simulink model "simLab11"  (R2023b)
settings: Solver=FixedStepAuto  StartTime=0.0  StopTime=100  FixedStep=0.01  RelTol=1e-3
values from neighbouring files (symbols this model uses):
  a1 = 1    [dcos.m]    (also in lab11.m = -1.95)
  a2 = -3.5    [dcos.m]    (also in lab11.m = 1.01)
  b0 = 1    [dcos.m]    (also in lab11.m = 0.5)
  kr = 0.7    [lab11.m]
  w = 1    [lab11.m]
settings Model: Creator=pc  LastModifiedBy=pc

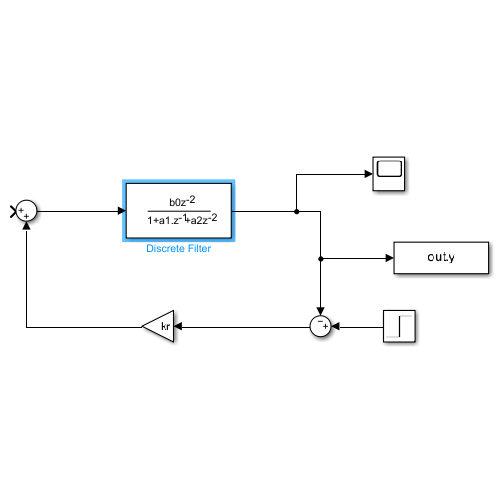
[thumbnail: Simulink's stored preview of the top-level diagram]
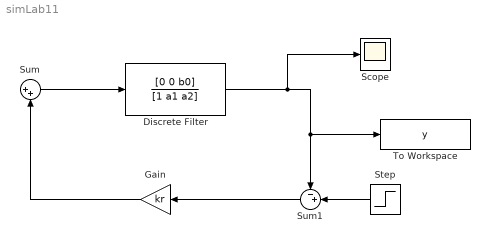
== system simLab11 ==
  Discrete Filter : DiscreteFilter  Numerator=[0 0 b0]  Denominator=[1 a1 a2]
  Gain : Gain  Gain=kr
  Scope : Scope
  Step : Step  Time=0  After=w  SampleTime=0
  Sum : Sum  Inputs=|++
  Sum1 : Sum  Inputs=-+|
  To Workspace : ToWorkspace  VariableName=y  SaveFormat=Timeseries  SampleTime=-1
  wires:
  Sum/1 -> Discrete Filter/1
  Discrete Filter/1 -> Scope/1, To Workspace/1, Sum1/1
  Step/1 -> Sum1/2
  Sum1/1 -> Gain/1
  Gain/1 -> Sum/2
